simulink model "Working_Shard"  (R2020b)
settings: Solver=VariableStepAuto  StartTime=0.0  StopTime=200  RelTol=1e-3
values from neighbouring files (symbols this model uses):
  A_2 = [0  0  0; 0  0  0; 0  0  0]    [Angular_gust.mat]    (also in Linear_gust.mat; Real_Values.m = zeros(3); Trial_Script.m = zeros(3); TryingNewAeroCoeffs.m = zeros(3))
  A_AD = [0 0 0 0 0 0 0 0 0 0 0 0 ... (36 elements, 6x6)]    [Angular_gust.mat]    (also in Linear_gust.mat; Real_Values.m = horzcat(A_i, A_ii); Trial_Script.m = horzcat(A_i, A_ii); TryingNewAeroCoeffs.m = horzcat(A_i, A_ii))
  A_kal = [0 0 0 0 0 0 0 0 0 0 0 0 ... (36 elements, 6x6)]    [Angular_gust.mat]    (also in Linear_gust.mat; Real_Values.m = [0 0 0 1 0 0; Trial_Script.m = [0 0 0 1 0 0; TryingNewAeroCoeffs.m = [0 0 0 1 0 0)
  B_2 = [0.0024294842205  2.57653534931e-06  6.44659625064e-05; 0  -0.000916808772026  -2.10833406567e-07; 0  0  -0.000799328564006]    [Angular_gust.mat]    (also in Linear_gust.mat; Real_Values.m = I_inv; Trial_Script.m = I_inv; TryingNewAeroCoeffs.m = I_inv)
  B_AD = [0 0 0 0 0 0 0 0 0 0 0 0 ... (36 elements, 6x6)]    [Angular_gust.mat]    (also in Linear_gust.mat; Real_Values.m = horzcat(B_i, B_ii); Trial_Script.m = horzcat(B_i, B_ii); TryingNewAeroCoeffs.m = horzcat(B_i, B_ii))
  B_kal = [0 0 0 0 0 0 0 0 0 0 0 0 ... (36 elements, 6x6)]    [Angular_gust.mat]    (also in Linear_gust.mat; Real_Values.m = [0 0 0 0 0 0; Trial_Script.m = [0 0 0 0 0 0; TryingNewAeroCoeffs.m = [0 0 0 0 0 0)
  C_2 = [1  0  0; 0  1  0; 0  0  1]    [Angular_gust.mat]    (also in Linear_gust.mat; Real_Values.m = eye(3); Trial_Script.m = eye(3); TryingNewAeroCoeffs.m = eye(3))
  C_AD = [1 0 0 0 0 0 0 1 0 0 0 0 ... (36 elements, 6x6)]    [Angular_gust.mat]    (also in Linear_gust.mat; Real_Values.m = eye(6); Trial_Script.m = eye(6); TryingNewAeroCoeffs.m = eye(6))
  C_D = 0.6    [Angular_gust.mat]    (also in Linear_gust.mat; Trial_Script.m; TryingNewAeroCoeffs.m)
  C_kal = [1 0 0 0 0 0 0 1 0 0 0 0 ... (36 elements, 6x6)]    [Angular_gust.mat]    (also in Linear_gust.mat; Real_Values.m = eye(6); Trial_Script.m = eye(6); TryingNewAeroCoeffs.m = eye(6))
  D_2 = [0  0  0; 0  0  0; 0  0  0]    [Angular_gust.mat]    (also in Linear_gust.mat; Real_Values.m = zeros(3); Trial_Script.m = zeros(3); TryingNewAeroCoeffs.m = zeros(3))
  D_AD = [0 0 0 0 0 0 0 0 0 0 0 0 ... (36 elements, 6x6)]    [Angular_gust.mat]    (also in Linear_gust.mat; Real_Values.m = zeros(6); Trial_Script.m = zeros(6); TryingNewAeroCoeffs.m = zeros(6))
  D_kal = [0 0 0 0 0 0 0 0 0 0 0 0 ... (36 elements, 6x6)]    [Angular_gust.mat]    (also in Linear_gust.mat; Real_Values.m = zeros(6); Trial_Script.m = zeros(6); TryingNewAeroCoeffs.m = zeros(6))
  delta_time = 0.0178961433409    [Angular_gust.mat]    (also in Linear_gust.mat; Real_Values.m = time/length(xdata); Trial_Script.m = time/length(xdata); TryingNewAeroCoeffs.m = time/length(xdata))
  Fb1_l = -2600    [Angular_gust.mat]    (also in Linear_gust.mat; Real_Values.m; Trial_Script.m; TryingNewAeroCoeffs.m)
  Fb1_u = 2600    [Angular_gust.mat]    (also in Linear_gust.mat; Real_Values.m; Trial_Script.m; TryingNewAeroCoeffs.m)
  Fb2_l = -2600    [Angular_gust.mat]    (also in Linear_gust.mat; Real_Values.m; Trial_Script.m; TryingNewAeroCoeffs.m)
  Fb2_u = 2600    [Angular_gust.mat]    (also in Linear_gust.mat; Real_Values.m; Trial_Script.m; TryingNewAeroCoeffs.m)
  Fb3_l = -3200    [Angular_gust.mat]    (also in Linear_gust.mat; Real_Values.m; Trial_Script.m; TryingNewAeroCoeffs.m)
  Fb3_u = 3200    [Angular_gust.mat]    (also in Linear_gust.mat; Real_Values.m; Trial_Script.m; TryingNewAeroCoeffs.m)
  Fb4_l = -3200    [Angular_gust.mat]    (also in Linear_gust.mat; Real_Values.m; Trial_Script.m; TryingNewAeroCoeffs.m)
  Fb4_u = 3200    [Angular_gust.mat]    (also in Linear_gust.mat; Real_Values.m; Trial_Script.m; TryingNewAeroCoeffs.m)
  Fc1_l = -300    [Angular_gust.mat]    (also in Linear_gust.mat; Real_Values.m = -30000; Trial_Script.m = -3000; TryingNewAeroCoeffs.m)
  Fc1_u = 300    [Angular_gust.mat]    (also in Linear_gust.mat; Real_Values.m = 30000; Trial_Script.m = 3000; TryingNewAeroCoeffs.m)
  Fc2_l = -300    [Angular_gust.mat]    (also in Linear_gust.mat; Real_Values.m = -30000; Trial_Script.m = -3000; TryingNewAeroCoeffs.m)
  Fc2_u = 300    [Angular_gust.mat]    (also in Linear_gust.mat; Real_Values.m = 30000; Trial_Script.m = 3000; TryingNewAeroCoeffs.m)
  Fc3_l = -300    [Angular_gust.mat]    (also in Linear_gust.mat; Real_Values.m = -30000; Trial_Script.m = -3000; TryingNewAeroCoeffs.m)
  Fc3_u = 300    [Angular_gust.mat]    (also in Linear_gust.mat; Real_Values.m = 30000; Trial_Script.m = 3000; TryingNewAeroCoeffs.m)
  Ft1_l = -5600    [Angular_gust.mat]    (also in Linear_gust.mat; Real_Values.m; Trial_Script.m; TryingNewAeroCoeffs.m)
  Ft1_u = 5600    [Angular_gust.mat]    (also in Linear_gust.mat; Real_Values.m; Trial_Script.m; TryingNewAeroCoeffs.m)
  Ft2_l = -5600    [Angular_gust.mat]    (also in Linear_gust.mat; Real_Values.m; Trial_Script.m; TryingNewAeroCoeffs.m)
  Ft2_u = 5600    [Angular_gust.mat]    (also in Linear_gust.mat; Real_Values.m; Trial_Script.m; TryingNewAeroCoeffs.m)
  Ft3_l = -3200    [Angular_gust.mat]    (also in Linear_gust.mat; Real_Values.m; Trial_Script.m; TryingNewAeroCoeffs.m)
  Ft3_u = 3200    [Angular_gust.mat]    (also in Linear_gust.mat; Real_Values.m; Trial_Script.m; TryingNewAeroCoeffs.m)
  Ft4_l = -3200    [Angular_gust.mat]    (also in Linear_gust.mat; Real_Values.m; Trial_Script.m; TryingNewAeroCoeffs.m)
  Ft4_u = 3200    [Angular_gust.mat]    (also in Linear_gust.mat; Real_Values.m; Trial_Script.m; TryingNewAeroCoeffs.m)
  g = 9.81    [Angular_gust.mat]    (also in Linear_gust.mat; Real_Values.m; Trial_Script.m; TryingNewAeroCoeffs.m)
  m = 941.102    [Angular_gust.mat]    (also in Linear_gust.mat; Real_Values.m; Trial_Script.m = 645; TryingNewAeroCoeffs.m)
  r_0 = [0 0 0]    [Angular_gust.mat]    (also in Linear_gust.mat; Real_Values.m = [0;0;0]; Trial_Script.m = [0;0;0]; TryingNewAeroCoeffs.m = [0;0;0])
  r_cgCatia = [0.0401998 0.00180957 -0.293434]    [Angular_gust.mat]    (also in Linear_gust.mat; Real_Values.m = TcgCatia*r_cgCatia; Trial_Script.m = [2; 0; 0]; TryingNewAeroCoeffs.m = TcgCatia*r_cgCatia)
  rho = 1.225    [Angular_gust.mat]    (also in Linear_gust.mat; Real_Values.m; Trial_Script.m; TryingNewAeroCoeffs.m)
  S = 1.8    [Angular_gust.mat]    (also in Linear_gust.mat; Trial_Script.m; TryingNewAeroCoeffs.m)
  t_finalgust = 17.9140394843    [Angular_gust.mat]    (also in Linear_gust.mat; Real_Values.m = time; TryingNewAeroCoeffs.m = time)
  TcgCatia = [1  0  0; 0  -1  0; 0  0  -1]    [Angular_gust.mat]    (also in Linear_gust.mat; Real_Values.m = [1 0 0; Trial_Script.m = [1 0 0; TryingNewAeroCoeffs.m = [1 0 0)
  theta_0 = [0 0 0]    [Angular_gust.mat]    (also in Linear_gust.mat; Real_Values.m = [0;0;0]; Trial_Script.m = [0;0;0]; TryingNewAeroCoeffs.m = [0;0;0])
  time_delay = 0.01    [Angular_gust.mat]    (also in Linear_gust.mat; Real_Values.m = 0.1; Trial_Script.m = 0.1; TryingNewAeroCoeffs.m)
  Tzy_Shard = [6.12323399574e-17  1  1.22464679915e-16; 1  -6.12323399574e-17  -7.49879891331e-33; 0  1.22464679915e-16  -1]    [Angular_gust.mat]    (also in Linear_gust.mat; Real_Values.m = [cos(pi/2) -sin(pi/2) 0; sin(pi/2) cos(pi/2) 0; 0 0 1]*[1 0 ; Trial_Script.m = [cos(pi/2) -sin(pi/2) 0; sin(pi/2) cos(pi/2) 0; 0 0 1]*[1 0 ; TryingNewAeroCoeffs.m = [cos(pi/2) -sin(pi/2) 0; sin(pi/2) cos(pi/2) 0; 0 0 1]*[1 0 )
  u0_final = 23.9559    [Angular_gust.mat]    (also in Linear_gust.mat; Real_Values.m = u_0(length(u_0)); TryingNewAeroCoeffs.m = u_0(length(u_0)))
  u1_final = -0.480858    [Angular_gust.mat]    (also in Linear_gust.mat; Real_Values.m = u_1(length(u_1)); TryingNewAeroCoeffs.m = u_1(length(u_1)))
  u2_final = -0.725589    [Angular_gust.mat]    (also in Linear_gust.mat; Real_Values.m = u_2(length(u_2)); TryingNewAeroCoeffs.m = u_2(length(u_2)))
  u_0 = [24.7775 24.7775 24.7775 24.7775 24.7775 24.7775 24.7775 24.7775 24.7775 24.7775 24.7775 24.7775 ... (1001 elements, 1001x1)]    [Angular_gust.mat]    (also in Linear_gust.mat; Real_Values.m = a(1:d_shard,1); Trial_Script.m = a(1:d_shard,1); TryingNewAeroCoeffs.m = a(1:d_shard,1))
  u_1 = [0.712897 0.712897 0.712897 0.712897 0.712897 0.712897 0.712897 0.712897 0.712897 0.712897 0.712897 0.712897 ... (1001 elements, 1001x1)]    [Angular_gust.mat]    (also in Linear_gust.mat; Real_Values.m = a(1:d_shard,2); Trial_Script.m = a(1:d_shard,2); TryingNewAeroCoeffs.m = a(1:d_shard,2))
  u_2 = [-0.504815 -0.504815 -0.504815 -0.504815 -0.504815 -0.504815 -0.504815 -0.504815 -0.504815 -0.504815 -0.504815 -0.504815 ... (1001 elements, 1001x1)]    [Angular_gust.mat]    (also in Linear_gust.mat; Real_Values.m = a(1:d_shard,3); Trial_Script.m = a(1:d_shard,3); TryingNewAeroCoeffs.m = a(1:d_shard,3))
  v_0 = [0 0 0]    [Angular_gust.mat]    (also in Linear_gust.mat; Real_Values.m = [0;0;0]; Trial_Script.m = [0;0;0]; TryingNewAeroCoeffs.m = [0;0;0])
  ZI_Cx = [4.10002314469 4.10486511138 4.10970707807 4.11454904475 4.11939101144 4.12423297813 4.12907494481 4.1339169115 4.13875887819 4.14360084487 4.14844281156 4.15328477825 ... (65341 elements, 361x181)]    [Angular_gust.mat]    (also in Linear_gust.mat; Real_Values.m = model_Cx(XI_Cx, YI_Cx); Trial_Script.m = model_Cx(XI_Cx, YI_Cx); TryingNewAeroCoeffs.m = model_Cx(XI_Cx, YI_Cx))
  ZI_Cy = [5.10662222372 5.15407485934 5.20152749496 5.24898013059 5.29643276621 5.34388540184 5.39133803746 5.43879067308 5.48624330871 5.53369594433 5.58114857996 5.62860121558 ... (65341 elements, 361x181)]    [Angular_gust.mat]    (also in Linear_gust.mat; Real_Values.m = model_Cy(XI_Cy, YI_Cy); Trial_Script.m = model_Cy(XI_Cy, YI_Cy); TryingNewAeroCoeffs.m = model_Cy(XI_Cy, YI_Cy))
  ZI_Cz = [-10.5947720774 -10.6317912004 -10.6688103235 -10.7058294465 -10.7428485695 -10.7798676926 -10.8168868156 -10.8539059387 -10.8909250617 -10.9279441847 -10.9649633078 -11.0019824308 ... (65341 elements, 361x181)]    [Angular_gust.mat]    (also in Linear_gust.mat; Real_Values.m = model_Cz(XI_Cz, YI_Cz); Trial_Script.m = model_Cz(XI_Cz, YI_Cz); TryingNewAeroCoeffs.m = model_Cz(XI_Cz, YI_Cz))
  ZI_p = [6.05111971338 6.06712776392 6.08313581446 6.099143865 6.11515191553 6.13115996607 6.14716801661 6.16317606715 6.17918411769 6.19519216823 6.21120021877 6.22720826931 ... (65341 elements, 361x181)]    [Angular_gust.mat]    (also in Linear_gust.mat; Real_Values.m = model_p(XI_p, YI_p); Trial_Script.m = model_p(XI_p, YI_p); TryingNewAeroCoeffs.m = model_p(XI_p, YI_p))
  ZI_q = [0.071083987219 0.054175962948 0.0372679386771 0.0203599144061 0.00345189013513 -0.0134561341358 -0.0303641584068 -0.0472721826778 -0.0641802069487 -0.0810882312197 -0.0979962554907 -0.114904279762 ... (65341 elements, 361x181)]    [Angular_gust.mat]    (also in Linear_gust.mat; Real_Values.m = model_q(XI_q, YI_q); Trial_Script.m = model_q(XI_q, YI_q); TryingNewAeroCoeffs.m = model_q(XI_q, YI_q))
  ZI_r = [-1.8762921931 -1.88364224017 -1.89099228723 -1.8983423343 -1.90569238136 -1.91304242842 -1.92039247549 -1.92774252255 -1.93509256961 -1.94244261668 -1.94979266374 -1.95714271081 ... (65341 elements, 361x181)]    [Angular_gust.mat]    (also in Linear_gust.mat; Real_Values.m = model_r(XI_r, YI_r); Trial_Script.m = model_r(XI_r, YI_r); TryingNewAeroCoeffs.m = model_r(XI_r, YI_r))
undefined symbols (not defined in the file or in its folder): Continuous, Time
libraries: dspsigops x11, simulink x7, pid_lib x3, fuzblock x3, dspindex x3, ctrlSharedLib x2, sharedutil x1, mpclib x1, dspmathops x1, cstblocks x1
(part 1 of 2)
settings Model: Creator=Jonathan van Zyl  LastModifiedBy=Jonathan van Zyl

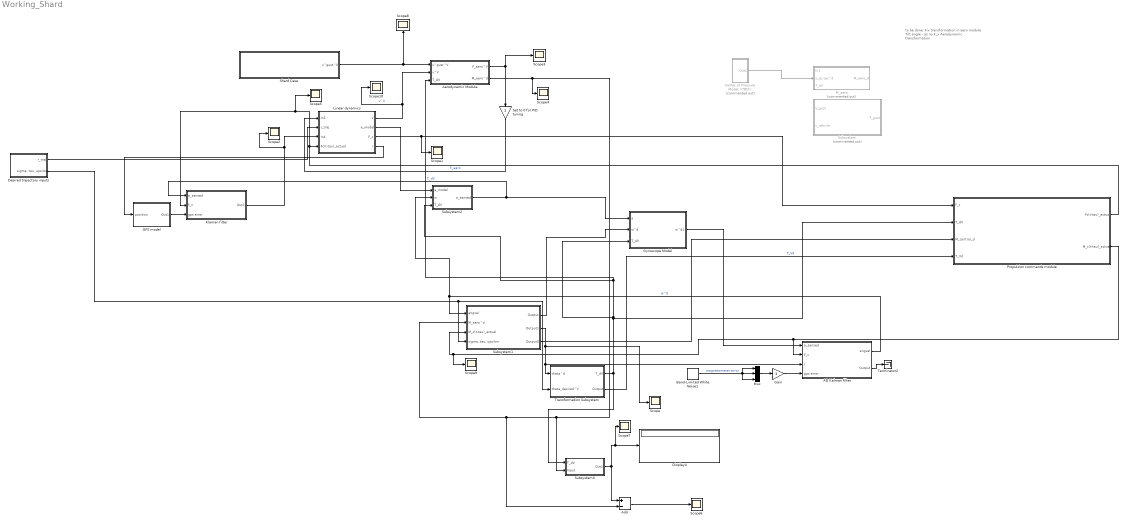
== system Working_Shard ==
  note: to be done:
      | Fix transformation in aero module
      | Tilt angle - as no F_x
      | Aerodynamic transformation
  AD Kalman filter : Subsystem
  Add : Sum  Inputs=+-
  Aerodynamic Module : Subsystem
  Band-Limited White Noise1 : simulink/Sources/Band-Limited White Noise  Cov=[0.000000001]  Ts=0.1  seed=[23341]
  Center of Pressure Model <TBD> : Subsystem  Commented=on
  Desired trajectory inputs : Subsystem
  Display4 : Display
  GPS model : Subsystem
  Gain : Gain
  Gyroscope Model : Subsystem
  Klaman filter : Subsystem
  Linear dynamics : Subsystem
  M_aero : Subsystem  Commented=on
  Mux : Mux  Inputs=3
  Propulsion commands module : Subsystem
  Scope{,1..10} (11 alike) : Scope
  Set to 0 for PID tuning : Gain
  Shard Case : Subsystem
  Subsystem : Subsystem  Commented=on
  Subsystem1 : Subsystem
  Subsystem2 : Subsystem
  Subsystem3 : Subsystem
  Terminator2 : Terminator
  Transformation Subsystem : Subsystem
  wires:
  Propulsion commands module/2(M_c(t-tau)_actual) -> AD Kalman filter/2(F_c), Scope9/1, Subsystem1/3(M_c(t-tau)_actual)
  Linear dynamics/3(F_c) -> Propulsion commands module/1(F_c), Scope1/1
  Gyroscope Model/1(w^d1) -> AD Kalman filter/1(a_sensed)
  GPS model/1(Out1) -> Klaman filter/3(gps error)
  Aerodynamic Module/2(M_aero^d) -> Scope4/1, Add/2, Subsystem1/2(M_aero^d), Subsystem3/2(Input)
  Subsystem3/1(Out1) -> Add/1, Scope7/1, Display4/1
  Shard Case/1(v^gust^V) -> Scope8/1, Aerodynamic Module/1(v^gust^V)
  Add/1 -> Scope6/1
  AD Kalman filter/1(angvel) -> Subsystem2/2(w), Subsystem1/1(angvel)  "w^d"
  Aerodynamic Module/1(F_aero^V) -> Set to 0 for PID tuning/1, Scope3/1
  Subsystem2/1(a_sensed) -> Gyroscope Model/1(a), Klaman filter/1(a_sensed)
  Linear dynamics/2(a_model) -> Subsystem2/1(a_model)
  Center of Pressure Model <TBD>/1(Out1) -> M_aero/2(x_cp vec^d)
  Subsystem1/2(Output1) -> Transformation Subsystem/1(theta^d), AD Kalman filter/3(r), Scope/1
  Transformation Subsystem/1(T_dV) -> Subsystem3/1(T_dV), Aerodynamic Module/3(T_dV), Subsystem2/3(T_dV), Gyroscope Model/3(T_dV), Propulsion commands module/2(T_dV)  "T_dV"
  Subsystem1/1(Output) -> Gyroscope Model/2(w^d)
  AD Kalman filter/2(Output) -> Terminator2/1
  Mux/1 -> Gain/1
  Gain/1 -> AD Kalman filter/4(gps error)
  Desired trajectory inputs/2("sigma, tau, upsilon") -> Transformation Subsystem/2(theta_desired^V), Subsystem1/4("sigma, tau, upsilon")
  Klaman filter/1(Out1) -> Scope2/1, Linear dynamics/3(In4)
  Desired trajectory inputs/1(r_traj) -> Linear dynamics/2(r_traj)
  Band-Limited White Noise1/1 -> Mux/1, Mux/2, Mux/3  "magnetometer error"
  Linear dynamics/1(v) -> Scope10/1, Aerodynamic Module/2(v^V)  "v^V"
  Subsystem1/3(Output3) -> Propulsion commands module/3(M_control_d)
  Linear dynamics/4(r) -> GPS model/1(position)
  Set to 0 for PID tuning/1 -> Linear dynamics/1(In1)  "F_aero"
  Propulsion commands module/1(Fc(t-tau)_actual) -> Scope5/1, Klaman filter/2(F_c), Linear dynamics/4(Fc(t-tau)_actual)
  Transformation Subsystem/2(Output) -> Propulsion commands module/4(T_Vd)  "T_Vd"

== system Working_Shard/AD Kalman filter ==
  a_sensed : Inport
  F_c : Inport  Port=2
  r : Inport  Port=3
  gps error : Inport  Port=4
  Add : Sum
  Constant4 : Constant  Value=0
  Demux1 : Demux  Outputs=6
  Gain4 : Gain
  Kalman Filter : ctrlSharedLib/Kalman Filter  TimeDomain=Continuous-Time  UseCurrentEstimator=on  ModelSource=Individual A, B, C, D matrices  ModelSourceVariable=ss(0.95,1,1,0,1)  A=A_AD  B=B_AD  C=C_AD  D=D_AD  NumberOfStates=1  NumberOfInputs=1  NumberOfOutputs=1  InitialEstimateSource=Dialog  X0=[0;0;0;0;0;0]  P0=10  UseK=off  UseGH=off  NumberOfProcessNoiseInputs=1  G=1  TimeInvariantG=on  H=0  TimeInvariantH=on  Q=0.05  TimeInvariantQ=on  R=1  TimeInvariantR=on  N=0  TimeInvariantN=on  AddInputPort=on  AddEnablePort=off  OutputEstimatedY=off  OutputP=off  Ts=-1
  Mux : Mux  Inputs=3
  Mux1 : Mux
  Mux2 : Mux  Inputs=2
  Mux3 : Mux  Inputs=3
  Scope1 : Scope
  angvel : Outport
  Output : Outport  Port=2
  wires:
  Demux1/5 -> Mux/2
  Mux2/1 -> Kalman Filter/2
  Constant4/1 -> Mux1/3, Mux1/1, Mux1/2
  gps error/1 -> Gain4/1  "theta_error"
  r/1 -> Scope1/1, Add/1  "theta_model"
  Demux1/4 -> Mux/1
  Demux1/2 -> Mux3/2
  Mux1/1 -> Kalman Filter/1
  F_c/1 -> Mux1/4  "Control Torques"
  Demux1/1 -> Mux3/1
  Kalman Filter/1 -> Demux1/1
  Demux1/6 -> Mux/3
  Gain4/1 -> Add/2
  Demux1/3 -> Mux3/3
  Add/1 -> Mux2/1  "theta_sensed"
  Mux3/1 -> angvel/1  "w_kalman"
  a_sensed/1 -> Mux2/2  "sensed angular velocity"
  Mux/1 -> Output/1  "wdot_kalman"

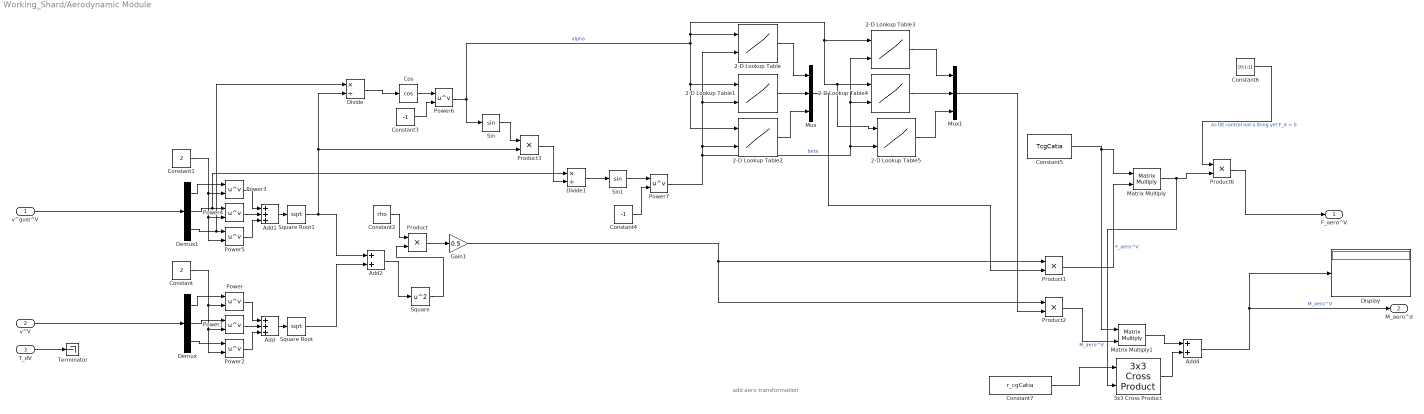
== system Working_Shard/Aerodynamic Module ==
  note: add aero transformation
  v^gust^V : Inport
  v^V : Inport  Port=2
  T_dV : Inport  Port=3
  2-D Lookup Table : Lookup_n-D  BreakpointsForDimension1=[-180:1:180]  BreakpointsForDimension2=[-180:1:180]  Table=ZI_Cx  InternalRulePriority=Speed  RndMeth=Simplest  InputSameDT=on
      settings: InputPortMap=u0,u1
  2-D Lookup Table1 : Lookup_n-D  BreakpointsForDimension1=[-180:1:180]  BreakpointsForDimension2=[-180:1:180]  Table=ZI_Cy  InternalRulePriority=Speed  RndMeth=Simplest  InputSameDT=on
      settings: InputPortMap=u0,u1
  2-D Lookup Table2 : Lookup_n-D  BreakpointsForDimension1=[-180:1:180]  BreakpointsForDimension2=[-180:1:180]  Table=ZI_Cz  InternalRulePriority=Speed  RndMeth=Simplest  InputSameDT=on
      settings: InputPortMap=u0,u1
  2-D Lookup Table3 : Lookup_n-D  BreakpointsForDimension1=[-180:1:180]  BreakpointsForDimension2=[-180:1:180]  Table=ZI_p  InternalRulePriority=Speed  RndMeth=Simplest  InputSameDT=on
      settings: InputPortMap=u0,u1
  2-D Lookup Table4 : Lookup_n-D  BreakpointsForDimension1=[-180:1:180]  BreakpointsForDimension2=[-180:1:180]  Table=ZI_q  InternalRulePriority=Speed  RndMeth=Simplest  InputSameDT=on
      settings: InputPortMap=u0,u1
  2-D Lookup Table5 : Lookup_n-D  BreakpointsForDimension1=[-180:1:180]  BreakpointsForDimension2=[-180:1:180]  Table=ZI_r  InternalRulePriority=Speed  RndMeth=Simplest  InputSameDT=on
      settings: InputPortMap=u0,u1
  3x3 Cross Product : sharedutil/3x3 Cross Product  aMode=aMode
      settings: SourceProductBaseCode=AE,PW,MT,UV,VE,VP
  Add : Sum  Inputs=+++
  Add1 : Sum  Inputs=+++
  Add2 : Sum
  Add4 : Sum
  Constant : Constant  Value=2
  Constant1 : Constant  Value=2
  Constant2 : Constant  Value=rho
  Constant3 : Constant  Value=-1
  Constant4 : Constant  Value=-1
  Constant5 : Constant  Value=TcgCatia
  Constant6 : Constant  Value=[0;1;1]
  Constant7 : Constant  Value=r_cgCatia
  Cos : Trigonometry  Operator=cos
  Demux : Demux  Outputs=3
  Demux1 : Demux  Outputs=3
  Display : Display
  Divide : Product  Inputs=*/
  Divide1 : Product  Inputs=*/
  Gain1 : Gain  Gain=0.5
  Matrix Multiply : Product  Multiplication=Matrix(*)
  Matrix Multiply1 : Product  Multiplication=Matrix(*)
  Mux : Mux  Inputs=3
  Mux1 : Mux  Inputs=3
  Power{,1..7} (8 alike) : Math  Operator=pow  SaturateOnIntegerOverflow=on
  Product{,1..3,6} (5 alike) : Product
  Sin : Trigonometry
  Sin1 : Trigonometry
  Square : Math  Operator=square  SaturateOnIntegerOverflow=on
  Square Root : Sqrt  SaturateOnIntegerOverflow=on
  Square Root1 : Sqrt  SaturateOnIntegerOverflow=on
  Terminator : Terminator
  F_aero^V : Outport
  M_aero^d : Outport  Port=2
  wires:
  Constant1/1 -> Power5/2, Power4/2, Power3/2
  Product1/1 -> Matrix Multiply/2  "F_aero^V"
  Square Root/1 -> Add2/2
  Power6/1 -> Sin/1, 2-D Lookup Table/1, 2-D Lookup Table5/1, 2-D Lookup Table4/1, 2-D Lookup Table3/1, 2-D Lookup Table2/1, 2-D Lookup Table1/1  "alpha"
  Power1/1 -> Add/2
  2-D Lookup Table5/1 -> Mux1/3
  Constant/1 -> Power2/2, Power1/2, Power/2
  Divide/1 -> Cos/1
  Demux/1 -> Power/1
  Power5/1 -> Add1/3
  2-D Lookup Table/1 -> Mux/1
  Divide1/1 -> Sin1/1
  Demux1/1 -> Power3/1
  Add2/1 -> Square/1
  Add4/1 -> Display/1, M_aero^d/1  "M_aero^V"
  Demux/3 -> Power2/1
  Constant4/1 -> Power7/2
  2-D Lookup Table4/1 -> Mux1/2
  Gain1/1 -> Product2/1, Product1/1
  Constant3/1 -> Power6/2
  Power7/1 -> 2-D Lookup Table/2, 2-D Lookup Table1/2, 2-D Lookup Table2/2, 2-D Lookup Table3/2, 2-D Lookup Table4/2, 2-D Lookup Table5/2  "beta"
  Cos/1 -> Power6/1
  Demux1/3 -> Divide/1, Power5/1
  Product/1 -> Gain1/1
  Sin1/1 -> Power7/1
  Power2/1 -> Add/3
  Sin/1 -> Product3/1
  Mux1/1 -> Product2/2
  Demux1/2 -> Divide1/1, Power4/1
  Power4/1 -> Add1/2
  Add/1 -> Square Root/1
  Power/1 -> Add/1
  Square Root1/1 -> Product3/2, Divide/2, Add2/1
  v^gust^V/1 -> Demux1/1
  2-D Lookup Table3/1 -> Mux1/1
  2-D Lookup Table1/1 -> Mux/2
  Power3/1 -> Add1/1
  Mux/1 -> Product1/2
  Product3/1 -> Divide1/2
  2-D Lookup Table2/1 -> Mux/3
  Add1/1 -> Square Root1/1
  Constant2/1 -> Product/1
  Demux/2 -> Power1/1
  v^V/1 -> Demux/1
  Square/1 -> Product/2
  Constant6/1 -> Product6/1  "As tilt control not a thing yet F_X = 0"
  Product6/1 -> F_aero^V/1
  T_dV/1 -> Terminator/1
  Constant5/1 -> Matrix Multiply1/1, Matrix Multiply/1
  Matrix Multiply/1 -> 3x3 Cross Product/2, Product6/2
  Constant7/1 -> 3x3 Cross Product/1
  Matrix Multiply1/1 -> Add4/1
  3x3 Cross Product/1 -> Add4/2
  Product2/1 -> Matrix Multiply1/2  "M_aero^V"

== system Working_Shard/Center of Pressure Model <TBD> ==
  Constant1 : Constant  Value=[0.1;0.2; 0.05]
  Out1 : Outport
  wires:
  Constant1/1 -> Out1/1  "x_cp"

== system Working_Shard/Desired trajectory inputs ==
  Constant2 : Constant  Value=[0;0; 0]
  Constant3 : Constant  Value=[0;0;0]
  r_traj : Outport
  "sigma, tau, upsilon" : Outport  Port=2
  wires:
  Constant2/1 -> r_traj/1  "r_traj"
  Constant3/1 -> "sigma, tau, upsilon"/1  "sigma, tau, upsilon"

== system Working_Shard/GPS model ==
  position : Inport
  GPS Model : MATLAB Function  TreatAsAtomicUnit=on
  Transpose : Math  Operator=transpose  SaturateOnIntegerOverflow=on
  Out1 : Outport
  wires:
  GPS Model/1(newposition) -> Transpose/1  "gps error"
  position/1 -> GPS Model/1(position)
  Transpose/1 -> Out1/1  "r_sensed"

== system Working_Shard/Gyroscope Model ==
  a : Inport
  w^d : Inport  Port=2
  T_dV : Inport  Port=3
  Demux : Demux  Outputs=3
  MATLAB Function : MATLAB Function  TreatAsAtomicUnit=on
  Terminator : Terminator
  Transpose : Math  Operator=transpose  SaturateOnIntegerOverflow=on
  Transpose2 : Math  Operator=transpose  SaturateOnIntegerOverflow=on
  w^d1 : Outport
  wires:
  T_dV/1 -> Terminator/1
  Transpose2/1 -> w^d1/1
  MATLAB Function/1(gyroData) -> Transpose2/1
  a/1 -> Transpose/1
  Transpose/1 -> MATLAB Function/4(acc)
  w^d/1 -> Demux/1
  Demux/1 -> MATLAB Function/1(xvel)
  Demux/2 -> MATLAB Function/2(yvel)
  Demux/3 -> MATLAB Function/3(zvel)

== system Working_Shard/Klaman filter ==
  a_sensed : Inport
  F_c : Inport  Port=2
  gps error : Inport  Port=3
  Constant4 : Constant  Value=0
  Demux1 : Demux  Outputs=6
  Integrator : Integrator  InitialCondition=v_0
  Kalman Filter : ctrlSharedLib/Kalman Filter  TimeDomain=Continuous-Time  UseCurrentEstimator=on  ModelSource=Individual A, B, C, D matrices  ModelSourceVariable=ss(0.95,1,1,0,1)  A=A_kal  B=B_kal  C=C_kal  D=D_kal  NumberOfStates=1  NumberOfInputs=1  NumberOfOutputs=1  InitialEstimateSource=Dialog  X0=[0;0;0;0;0;0]  P0=10  UseK=off  UseGH=off  NumberOfProcessNoiseInputs=1  G=1  TimeInvariantG=on  H=0  TimeInvariantH=on  Q=0.05  TimeInvariantQ=on  R=1  TimeInvariantR=on  N=0  TimeInvariantN=on  AddInputPort=on  AddEnablePort=off  OutputEstimatedY=off  OutputP=off  Ts=-1
  Mux1 : Mux
  Mux2 : Mux  Inputs=2
  Mux3 : Mux  Inputs=3
  Terminator : Terminator
  Terminator1 : Terminator
  Terminator2 : Terminator
  Out1 : Outport
  wires:
  Demux1/5 -> Terminator1/1
  Mux2/1 -> Kalman Filter/2
  Constant4/1 -> Mux1/3, Mux1/1, Mux1/2
  Demux1/4 -> Terminator/1
  Demux1/2 -> Mux3/2
  Mux1/1 -> Kalman Filter/1
  F_c/1 -> Mux1/4  "Control Force"
  Demux1/1 -> Mux3/1
  Kalman Filter/1 -> Demux1/1
  Demux1/6 -> Terminator2/1
  Demux1/3 -> Mux3/3
  Integrator/1 -> Mux2/2  "v_sensed"
  gps error/1 -> Mux2/1  "r_sensed"
  Mux3/1 -> Out1/1  "r_kalman"
  a_sensed/1 -> Integrator/1  "sensed acceleration"

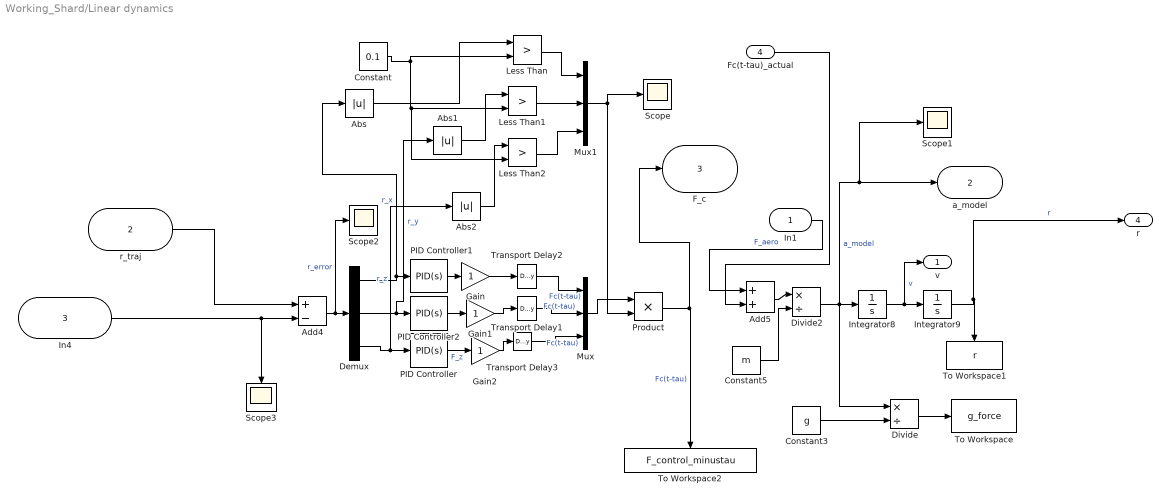
== system Working_Shard/Linear dynamics ==
  In1 : Inport
  r_traj : Inport  Port=2
  In4 : Inport  Port=3
  Fc(t-tau)_actual : Inport  Port=4
  Abs : Abs
  Abs1 : Abs
  Abs2 : Abs
  Add4 : Sum  Inputs=+-
  Add5 : Sum
  Constant : Constant  Value=0.1
  Constant3 : Constant  Value=g
  Constant5 : Constant  Value=m
  Demux : Demux  Outputs=3
  Divide : Product  Inputs=*/
  Divide2 : Product  Inputs=*/
  Gain : Gain
  Gain1 : Gain
  Gain2 : Gain
  Integrator8 : Integrator  InitialCondition=[0;0;0]
  Integrator9 : Integrator  InitialCondition=r_0
  Less Than : RelationalOperator  Operator=>  OutDataTypeStr=boolean  RndMeth=Simplest
  Less Than1 : RelationalOperator  Operator=>  OutDataTypeStr=boolean  RndMeth=Simplest
  Less Than2 : RelationalOperator  Operator=>  OutDataTypeStr=boolean  RndMeth=Simplest
  Mux : Mux  Inputs=3
  Mux1 : Mux  Inputs=3
  PID Controller : pid_lib/PID Controller  Controller=PID  Form=Parallel  TimeDomain=Continuous-time  UseExternalTs=off  SampleTime=-1  IntegratorMethod=Forward Euler  FilterMethod=Forward Euler  ControllerParametersSource=internal  P=9009.63914576468  I=3464.3602040453  D=5659.73322598295  UseFilter=on  N=27.0214258529072  TunerSelectOption=Transfer Function Based (PID Tuner App)  InitialConditionSource=internal  InitialConditionForIntegrator=0  InitialConditionForFilter=0  DifferentiatorICPrevScaledInput=0  ExternalReset=none  TrackingMode=off  Kt=1  LimitOutput=off  SatLimitsSource=internal  UpperSaturationLimit=inf  LowerSaturationLimit=-inf  LinearizeAsGain=on  AntiWindupMode=none  Kb=1  POutMin=[]  POutMax=[]  IOutMin=[]  IOutMax=[]  DOutMin=[]  DOutMax=[]  NOutMin=[]  NOutMax=[]  SumOutMin=[]  SumOutMax=[]  SaturationOutMin=[]  SaturationOutMax=[]  PParamMin=[]  PParamMax=[]  IParamMin=[]  IParamMax=[]  DParamMin=[]  DParamMax=[]  NParamMin=[]  NParamMax=[]  KbParamMin=[]  KbParamMax=[]  KtParamMin=[]  KtParamMax=[]  KbOutMin=[]  KbOutMax=[]  KtOutMin=[]  KtOutMax=[]  IntegratorOutMin=[]  IntegratorOutMax=[]  FilterOutMin=[]  FilterOutMax=[]  SumI1OutMin=[]  SumI1OutMax=[]  SumI2OutMin=[]  SumI2OutMax=[]  SumI3OutMin=[]  SumI3OutMax=[]  SumI4OutMin=[]  SumI4OutMax=[]  SumDOutMin=[]  SumDOutMax=[]  DifferentiatorOutMin=[]  DifferentiatorOutMax=[]  FilterDiffOutCoefMin=[]  FilterDiffOutCoefMax=[]  ReciprocalOutMin=[]  ReciprocalOutMax=[]  SumDenOutMin=[]  SumDenOutMax=[]  SumNumOutMin=[]  SumNumOutMax=[]  DivideOutMin=[]  DivideOutMax=[]  UdiffTsProdOutMin=[]  UdiffTsProdOutMax=[]  NTsProdOutMin=[]  NTsProdOutMax=[]  UintegralTsProdOutMin=[]  UintegralTsProdOutMax=[]  UngainTsProdOutMin=[]  UngainTsProdOutMax=[]  IntegratorContinuousStateAttributes=''  IntegratorStateMustResolveToSignalObject=off  IntegratorRTWStateStorageClass=Auto  FilterContinuousStateAttributes=''  FilterStateMustResolveToSignalObject=off  FilterRTWStateStorageClass=Auto  ParallelPVariant=InternalParameters  IdealPVariant=Disabled  IVariant=InternalParameters  DVariant=InternalParameters  IntegratorVariant=Continuous  SatVariant=Disabled  AWVariant=Passthrough  PCopyVariant=Disabled  TRVariant=Disabled  FdbkBlocksVariant=Forward  IdealPFdbkVariant=Disabled  SatFdbkVariant=Disabled  DerivativeFilterVariant=ContFilter  NVariant=InternalParameters  NCopyVariant=Disabled  FilterICVariant=InternalICsFilter  IntegratorICVariant=InternalICs  ExternalResetVariant=Disabled  TRSumVariant=Passthrough  SumFdbkVariant=Disabled  SumVariant=Sum_PID  TsampFilterVariant=InternalTs  TsampNgainVariant=Passthrough  TsampIntegralVariant=Passthrough  ExternalSaturationOutDataTypeStr=Inherit: Same as second input
  PID Controller1 : pid_lib/PID Controller  Controller=PID  Form=Parallel  TimeDomain=Continuous-time  UseExternalTs=off  SampleTime=-1  IntegratorMethod=Forward Euler  FilterMethod=Forward Euler  ControllerParametersSource=internal  P=9009.63914576468  I=3464.36020404063  D=5659.73322596604  UseFilter=on  N=27.0214258528983  TunerSelectOption=Transfer Function Based (PID Tuner App)  InitialConditionSource=internal  InitialConditionForIntegrator=0  InitialConditionForFilter=0  DifferentiatorICPrevScaledInput=0  ExternalReset=none  TrackingMode=off  Kt=1  LimitOutput=off  SatLimitsSource=internal  UpperSaturationLimit=inf  LowerSaturationLimit=-inf  LinearizeAsGain=on  AntiWindupMode=none  Kb=1  POutMin=[]  POutMax=[]  IOutMin=[]  IOutMax=[]  DOutMin=[]  DOutMax=[]  NOutMin=[]  NOutMax=[]  SumOutMin=[]  SumOutMax=[]  SaturationOutMin=[]  SaturationOutMax=[]  PParamMin=[]  PParamMax=[]  IParamMin=[]  IParamMax=[]  DParamMin=[]  DParamMax=[]  NParamMin=[]  NParamMax=[]  KbParamMin=[]  KbParamMax=[]  KtParamMin=[]  KtParamMax=[]  KbOutMin=[]  KbOutMax=[]  KtOutMin=[]  KtOutMax=[]  IntegratorOutMin=[]  IntegratorOutMax=[]  FilterOutMin=[]  FilterOutMax=[]  SumI1OutMin=[]  SumI1OutMax=[]  SumI2OutMin=[]  SumI2OutMax=[]  SumI3OutMin=[]  SumI3OutMax=[]  SumI4OutMin=[]  SumI4OutMax=[]  SumDOutMin=[]  SumDOutMax=[]  DifferentiatorOutMin=[]  DifferentiatorOutMax=[]  FilterDiffOutCoefMin=[]  FilterDiffOutCoefMax=[]  ReciprocalOutMin=[]  ReciprocalOutMax=[]  SumDenOutMin=[]  SumDenOutMax=[]  SumNumOutMin=[]  SumNumOutMax=[]  DivideOutMin=[]  DivideOutMax=[]  UdiffTsProdOutMin=[]  UdiffTsProdOutMax=[]  NTsProdOutMin=[]  NTsProdOutMax=[]  UintegralTsProdOutMin=[]  UintegralTsProdOutMax=[]  UngainTsProdOutMin=[]  UngainTsProdOutMax=[]  IntegratorContinuousStateAttributes=''  IntegratorStateMustResolveToSignalObject=off  IntegratorRTWStateStorageClass=Auto  FilterContinuousStateAttributes=''  FilterStateMustResolveToSignalObject=off  FilterRTWStateStorageClass=Auto  ParallelPVariant=InternalParameters  IdealPVariant=Disabled  IVariant=InternalParameters  DVariant=InternalParameters  IntegratorVariant=Continuous  SatVariant=Disabled  AWVariant=Passthrough  PCopyVariant=Disabled  TRVariant=Disabled  FdbkBlocksVariant=Forward  IdealPFdbkVariant=Disabled  SatFdbkVariant=Disabled  DerivativeFilterVariant=ContFilter  NVariant=InternalParameters  NCopyVariant=Disabled  FilterICVariant=InternalICsFilter  IntegratorICVariant=InternalICs  ExternalResetVariant=Disabled  TRSumVariant=Passthrough  SumFdbkVariant=Disabled  SumVariant=Sum_PID  TsampFilterVariant=InternalTs  TsampNgainVariant=Passthrough  TsampIntegralVariant=Passthrough  ExternalSaturationOutDataTypeStr=Inherit: Same as second input
  PID Controller2 : pid_lib/PID Controller  Controller=PID  Form=Parallel  TimeDomain=Continuous-time  UseExternalTs=off  SampleTime=-1  IntegratorMethod=Forward Euler  FilterMethod=Forward Euler  ControllerParametersSource=internal  P=9009.63914576468  I=3464.36020397681  D=5659.73322587286  UseFilter=on  N=27.0214258527793  TunerSelectOption=Transfer Function Based (PID Tuner App)  InitialConditionSource=internal  InitialConditionForIntegrator=0  InitialConditionForFilter=0  DifferentiatorICPrevScaledInput=0  ExternalReset=none  TrackingMode=off  Kt=1  LimitOutput=off  SatLimitsSource=internal  UpperSaturationLimit=inf  LowerSaturationLimit=-inf  LinearizeAsGain=on  AntiWindupMode=none  Kb=1  POutMin=[]  POutMax=[]  IOutMin=[]  IOutMax=[]  DOutMin=[]  DOutMax=[]  NOutMin=[]  NOutMax=[]  SumOutMin=[]  SumOutMax=[]  SaturationOutMin=[]  SaturationOutMax=[]  PParamMin=[]  PParamMax=[]  IParamMin=[]  IParamMax=[]  DParamMin=[]  DParamMax=[]  NParamMin=[]  NParamMax=[]  KbParamMin=[]  KbParamMax=[]  KtParamMin=[]  KtParamMax=[]  KbOutMin=[]  KbOutMax=[]  KtOutMin=[]  KtOutMax=[]  IntegratorOutMin=[]  IntegratorOutMax=[]  FilterOutMin=[]  FilterOutMax=[]  SumI1OutMin=[]  SumI1OutMax=[]  SumI2OutMin=[]  SumI2OutMax=[]  SumI3OutMin=[]  SumI3OutMax=[]  SumI4OutMin=[]  SumI4OutMax=[]  SumDOutMin=[]  SumDOutMax=[]  DifferentiatorOutMin=[]  DifferentiatorOutMax=[]  FilterDiffOutCoefMin=[]  FilterDiffOutCoefMax=[]  ReciprocalOutMin=[]  ReciprocalOutMax=[]  SumDenOutMin=[]  SumDenOutMax=[]  SumNumOutMin=[]  SumNumOutMax=[]  DivideOutMin=[]  DivideOutMax=[]  UdiffTsProdOutMin=[]  UdiffTsProdOutMax=[]  NTsProdOutMin=[]  NTsProdOutMax=[]  UintegralTsProdOutMin=[]  UintegralTsProdOutMax=[]  UngainTsProdOutMin=[]  UngainTsProdOutMax=[]  IntegratorContinuousStateAttributes=''  IntegratorStateMustResolveToSignalObject=off  IntegratorRTWStateStorageClass=Auto  FilterContinuousStateAttributes=''  FilterStateMustResolveToSignalObject=off  FilterRTWStateStorageClass=Auto  ParallelPVariant=InternalParameters  IdealPVariant=Disabled  IVariant=InternalParameters  DVariant=InternalParameters  IntegratorVariant=Continuous  SatVariant=Disabled  AWVariant=Passthrough  PCopyVariant=Disabled  TRVariant=Disabled  FdbkBlocksVariant=Forward  IdealPFdbkVariant=Disabled  SatFdbkVariant=Disabled  DerivativeFilterVariant=ContFilter  NVariant=InternalParameters  NCopyVariant=Disabled  FilterICVariant=InternalICsFilter  IntegratorICVariant=InternalICs  ExternalResetVariant=Disabled  TRSumVariant=Passthrough  SumFdbkVariant=Disabled  SumVariant=Sum_PID  TsampFilterVariant=InternalTs  TsampNgainVariant=Passthrough  TsampIntegralVariant=Passthrough  ExternalSaturationOutDataTypeStr=Inherit: Same as second input
  Product : Product
  Scope{,1..3} (4 alike) : Scope
  To Workspace : ToWorkspace  VariableName=g_force  SaveFormat=Timeseries  SampleTime=-1
      settings: Save2DSignal=2-D array (concatenate along first dimension)
  To Workspace1 : ToWorkspace  VariableName=r  SaveFormat=Timeseries  SampleTime=-1
  To Workspace2 : ToWorkspace  VariableName=F_control_minustau  SaveFormat=Timeseries  SampleTime=-1
  Transport Delay1 : TransportDelay  DelayTime=time_delay  TransDelayFeedthrough=on
  Transport Delay2 : TransportDelay  DelayTime=time_delay  TransDelayFeedthrough=on
  Transport Delay3 : TransportDelay  DelayTime=time_delay  TransDelayFeedthrough=on
  v : Outport
  a_model : Outport  Port=2
  F_c : Outport  Port=3
  r : Outport  Port=4
  wires:
  Divide2/1 -> Divide/1, Scope1/1, a_model/1, Integrator8/1  "a_model"
  In4/1 -> Add4/2, Scope3/1
  Divide/1 -> To Workspace/1
  r_traj/1 -> Add4/1
  PID Controller2/1 -> Gain1/1
  Add5/1 -> Divide2/1
  Constant5/1 -> Divide2/2
  Demux/1 -> Abs/1, PID Controller1/1  "r_x"
  PID Controller/1 -> Gain2/1  "F_z"
  Gain1/1 -> Transport Delay1/1
  Add4/1 -> Scope2/1, Demux/1  "r_error"
  Integrator9/1 -> r/1, To Workspace1/1  "r"
  Demux/2 -> Abs1/1, PID Controller2/1  "r_y"
  Product/1 -> F_c/1, To Workspace2/1  "Fc(t-tau)"
  PID Controller1/1 -> Gain/1
  Constant3/1 -> Divide/2
  Gain/1 -> Transport Delay2/1
  Demux/3 -> Abs2/1, PID Controller/1  "r_z"
  Gain2/1 -> Transport Delay3/1
  Integrator8/1 -> Integrator9/1, v/1  "v"
  In1/1 -> Add5/1  "F_aero"
  Transport Delay2/1 -> Mux/1  "Fc(t-tau)"
  Transport Delay1/1 -> Mux/2  "Fc(t-tau)"
  Transport Delay3/1 -> Mux/3  "Fc(t-tau)"
  Constant/1 -> Less Than2/2, Less Than1/2, Less Than/2
  Less Than1/1 -> Mux1/2
  Less Than/1 -> Mux1/1
  Less Than2/1 -> Mux1/3
  Mux/1 -> Product/1
  Mux1/1 -> Product/2, Scope/1
  Abs/1 -> Less Than/1
  Abs1/1 -> Less Than1/1
  Abs2/1 -> Less Than2/1
  Fc(t-tau)_actual/1 -> Add5/2

== system Working_Shard/M_aero ==
  In1 : Inport
  x_cp vec^d : Inport  Port=2
  T_dV : Inport  Port=3
  Matrix Multiply : Product  Multiplication=Matrix(*)
  Matrix Multiply1 : Product
  M_aero_d : Outport
  wires:
  Matrix Multiply/1 -> Matrix Multiply1/2  "F_dis^d"
  x_cp vec^d/1 -> Matrix Multiply1/1  "x_cp"
  T_dV/1 -> Matrix Multiply/1
  In1/1 -> Matrix Multiply/2  "F_gust"
  Matrix Multiply1/1 -> M_aero_d/1  "M_aero_d"

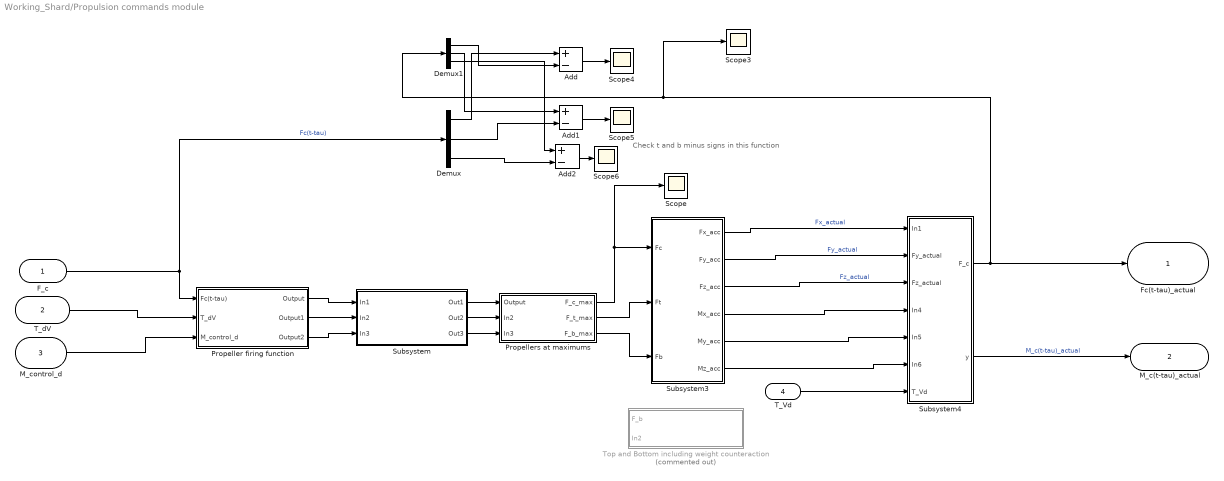
== system Working_Shard/Propulsion commands module ==
  note: Check t and b minus signs in this function
  F_c : Inport
  T_dV : Inport  Port=2
  M_control_d : Inport  Port=3
  T_Vd : Inport  Port=4
  Add : Sum  Inputs=+-
  Add1 : Sum  Inputs=+-
  Add2 : Sum  Inputs=+-
  Demux : Demux  Outputs=3
  Demux1 : Demux  Outputs=3
  Propeller firing function : Subsystem
  Propellers at maximums : Subsystem
  Scope{,3..6} (5 alike) : Scope
  Subsystem : Subsystem
  Subsystem3 : Subsystem
  Subsystem4 : Subsystem
  Top and Bottom including weight counteraction : Subsystem  Commented=on
  Fc(t-tau)_actual : Outport
  M_c(t-tau)_actual : Outport  Port=2
  wires:
  Subsystem3/2(Fy_acc) -> Subsystem4/2(Fy_actual)  "Fy_actual"
  Subsystem4/1(F_c) -> Fc(t-tau)_actual/1, Scope3/1, Demux1/1
  Demux1/3 -> Add2/1
  Subsystem3/3(Fz_acc) -> Subsystem4/3(Fz_actual)  "Fz_actual"
  Demux/2 -> Add1/2
  T_dV/1 -> Propeller firing function/2(T_dV)
  Subsystem3/1(Fx_acc) -> Subsystem4/1(In1)  "Fx_actual"
  Demux1/2 -> Add1/1
  Propellers at maximums/2(F_t_max) -> Subsystem3/2(Ft)
  Demux1/1 -> Add/2
  Subsystem3/5(My_acc) -> Subsystem4/5(In5)
  Subsystem3/6(Mz_acc) -> Subsystem4/6(In6)
  Propellers at maximums/3(F_b_max) -> Subsystem3/3(Fb)
  Demux/3 -> Add2/2
  Subsystem4/2(y) -> M_c(t-tau)_actual/1  "M_c(t-tau)_actual"
  F_c/1 -> Demux/1, Propeller firing function/1(Fc(t-tau))  "Fc(t-tau)"
  T_Vd/1 -> Subsystem4/7(T_Vd)
  Subsystem3/4(Mx_acc) -> Subsystem4/4(In4)
  Add1/1 -> Scope5/1
  Propellers at maximums/1(F_c_max) -> Scope/1, Subsystem3/1(Fc)
  Add2/1 -> Scope6/1
  Demux/1 -> Add/1
  Add/1 -> Scope4/1
  M_control_d/1 -> Propeller firing function/3(M_control_d)
  Propeller firing function/1(Output) -> Subsystem/1(In1)
  Propeller firing function/2(Output1) -> Subsystem/2(In2)
  Propeller firing function/3(Output2) -> Subsystem/3(In3)
  Subsystem/1(Out1) -> Propellers at maximums/1(Output)
  Subsystem/2(Out2) -> Propellers at maximums/2(In2)
  Subsystem/3(Out3) -> Propellers at maximums/3(In3)

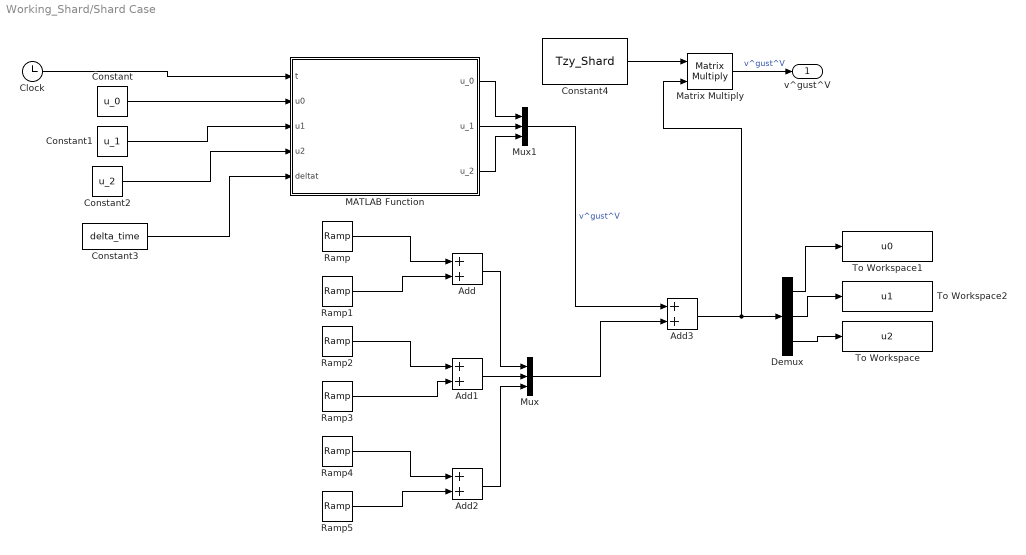
== system Working_Shard/Shard Case ==
  Add{,1..3} (4 alike) : Sum
  Clock : Clock
  Constant : Constant  Value=u_0
  Constant1 : Constant  Value=u_1
  Constant2 : Constant  Value=u_2
  Constant3 : Constant  Value=delta_time
  Constant4 : Constant  Value=Tzy_Shard
  Demux : Demux  Outputs=3
  MATLAB Function : MATLAB Function  TreatAsAtomicUnit=on
  Matrix Multiply : Product  Multiplication=Matrix(*)
  Mux : Mux  Inputs=3
  Mux1 : Mux  Inputs=3
  Ramp : simulink/Sources/Ramp  slope=-1  start=t_finalgust  InitialOutput=0
  Ramp1 : simulink/Sources/Ramp  slope=1  start=t_finalgust + u0_final  InitialOutput=0
  Ramp2 : simulink/Sources/Ramp  slope=-1  start=t_finalgust  InitialOutput=0
  Ramp3 : simulink/Sources/Ramp  slope=1  start=t_finalgust + u1_final  InitialOutput=0
  Ramp4 : simulink/Sources/Ramp  slope=-1  start=t_finalgust  InitialOutput=0
  Ramp5 : simulink/Sources/Ramp  slope=1  start=t_finalgust + u2_final  InitialOutput=0
  To Workspace : ToWorkspace  VariableName=u2  SaveFormat=Timeseries  SampleTime=-1
  To Workspace1 : ToWorkspace  VariableName=u0  SaveFormat=Timeseries  SampleTime=-1
  To Workspace2 : ToWorkspace  VariableName=u1  SaveFormat=Timeseries  SampleTime=-1
  v^gust^V : Outport
  wires:
  Constant2/1 -> MATLAB Function/4(u2)
  Clock/1 -> MATLAB Function/1(t)
  Constant4/1 -> Matrix Multiply/1
  Constant1/1 -> MATLAB Function/3(u1)
  MATLAB Function/2(u_1) -> Mux1/2
  MATLAB Function/3(u_2) -> Mux1/3
  MATLAB Function/1(u_0) -> Mux1/1
  Constant/1 -> MATLAB Function/2(u0)
  Constant3/1 -> MATLAB Function/5(deltat)
  Mux1/1 -> Add3/1  "v^gust^V"
  Matrix Multiply/1 -> v^gust^V/1  "v^gust^V"
  Ramp/1 -> Add/1
  Ramp1/1 -> Add/2
  Ramp3/1 -> Add1/2
  Ramp2/1 -> Add1/1
  Ramp5/1 -> Add2/2
  Ramp4/1 -> Add2/1
  Add/1 -> Mux/1
  Add1/1 -> Mux/2
  Add2/1 -> Mux/3
  Mux/1 -> Add3/2
  Add3/1 -> Demux/1, Matrix Multiply/2
  Demux/2 -> To Workspace2/1
  Demux/3 -> To Workspace/1
  Demux/1 -> To Workspace1/1

== system Working_Shard/Subsystem ==
  V_gust : Inport
  v_vehicle : Inport  Port=2
  Add2 : Sum
  Add3 : Sum
  Drag1 : Subsystem
  Product : Product
  Scope : Scope
  Step2 : Step  Time=0  SampleTime=0
  Step3 : Step  Time=10.5  After=-1  SampleTime=0
  To Workspace : ToWorkspace  VariableName=v_sumsq  SampleTime=-1
  To Workspace1 : ToWorkspace  VariableName=step  SaveFormat=Timeseries  SampleTime=-1
  To Workspace2 : ToWorkspace  VariableName=vtotal  SaveFormat=Timeseries  SampleTime=-1
  To Workspace3 : ToWorkspace  VariableName=F_gust  SaveFormat=Timeseries  SampleTime=-1
  To Workspace4 : ToWorkspace  VariableName=v_gust  SaveFormat=Timeseries  SampleTime=-1
  F_gust : Outport
  wires:
  Product/1 -> F_gust/1, To Workspace3/1, Scope/1  "F_gust"
  Step3/1 -> Add2/1
  V_gust/1 -> To Workspace4/1, Add3/1
  Drag1/1(Out1) -> To Workspace/1
  Add3/1 -> Drag1/1(In1), To Workspace2/1
  Add2/1 -> To Workspace1/1, Product/2
  Step2/1 -> Add2/2
  v_vehicle/1 -> Add3/2
  Drag1/2(drag) -> Product/1

== system Working_Shard/Subsystem1 ==
  angvel : Inport
  M_aero^d : Inport  Port=2
  M_c(t-tau)_actual : Inport  Port=3
  "sigma, tau, upsilon" : Inport  Port=4
  Subsystem : Subsystem
  Output : Outport
  Output1 : Outport  Port=2
  Output3 : Outport  Port=3
  wires:
  M_aero^d/1 -> Subsystem/1(M_aero^d)  "M_aero^d"
  "sigma, tau, upsilon"/1 -> Subsystem/2(Input)  "sigma, tau upsilon"
  Subsystem/1(Output) -> Output1/1  "theta^d"
  Subsystem/2(Output1) -> Output3/1
  Subsystem/3(Out1) -> Output/1
  angvel/1 -> Subsystem/3(angvel)  "angelvel"
  M_c(t-tau)_actual/1 -> Subsystem/4(M_c(t-tau)_actual)

== system Working_Shard/Subsystem2 ==
  a_model : Inport
  w : Inport  Port=2
  T_dV : Inport  Port=3
  Display : Display
  Display1 : Display
  MATLAB Function : MATLAB Function  Commented=on  TreatAsAtomicUnit=on
  Terminator : Terminator
  Terminator3 : Terminator
  Transpose : Math  Operator=transpose  SaturateOnIntegerOverflow=on
  Transpose1 : Math  Operator=transpose  SaturateOnIntegerOverflow=on
  Transpose2 : Math  Operator=transpose  SaturateOnIntegerOverflow=on
  a_sensed : Outport
  wires:
  T_dV/1 -> Terminator3/1
  a_model/1 -> Transpose1/1
  Transpose2/1 -> a_sensed/1  "a_sensed"
  w/1 -> Transpose/1
  Transpose/1 -> Terminator/1
  Transpose1/1 -> Display1/1, Transpose2/1, Display/1  "a_sensed"

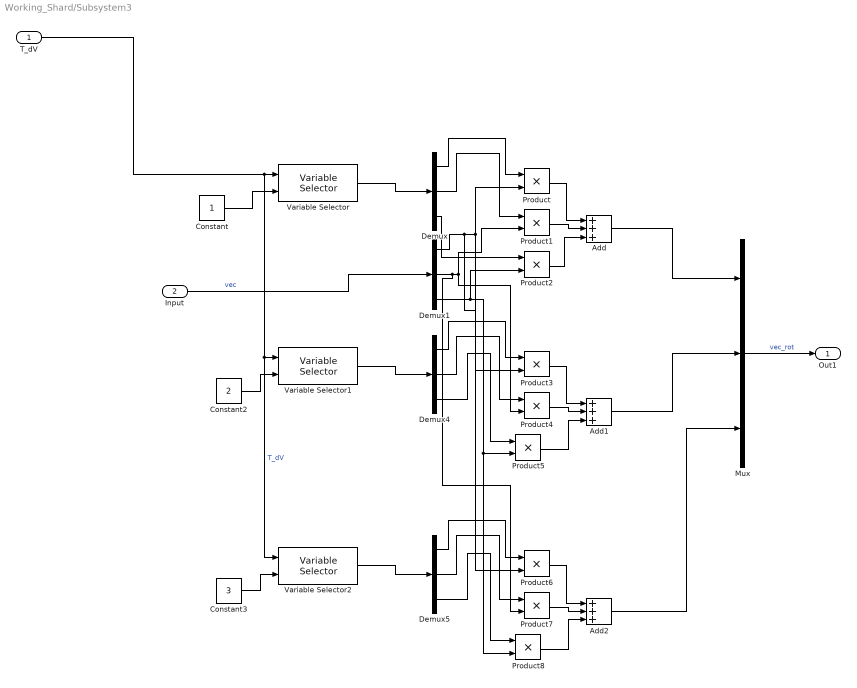
== system Working_Shard/Subsystem3 ==
  T_dV : Inport
  Input : Inport  Port=2
  Add : Sum  Inputs=+++
  Add1 : Sum  Inputs=+++
  Add2 : Sum  Inputs=+++
  Constant : Constant
  Constant2 : Constant  Value=2
  Constant3 : Constant  Value=3
  Demux{,1,4..5} (4 alike) : Demux  Outputs=3
  Mux : Mux  Inputs=3
  Product{,1..8} (9 alike) : Product
  Variable Selector : dspindex/Variable Selector  NumInputs=1  rowsOrCols=Columns  IdxMode=Variable  Elements=[1 3]  ZerOneIdxMode=One-based  errmode=Clip Index  FillMode=on  FillValues=0
  Variable Selector1 : dspindex/Variable Selector  NumInputs=1  rowsOrCols=Columns  IdxMode=Variable  Elements=[1 3]  ZerOneIdxMode=One-based  errmode=Clip Index  FillMode=on  FillValues=0
  Variable Selector2 : dspindex/Variable Selector  NumInputs=1  rowsOrCols=Columns  IdxMode=Variable  Elements=[1 3]  ZerOneIdxMode=One-based  errmode=Clip Index  FillMode=on  FillValues=0
  Out1 : Outport
  wires:
  Variable Selector/1 -> Demux/1
  Add2/1 -> Mux/3
  Demux/1 -> Product/1
  Product3/1 -> Add1/1
  Variable Selector1/1 -> Demux4/1
  Product4/1 -> Add1/2
  Demux4/2 -> Product4/1
  Demux/2 -> Product1/1
  Constant2/1 -> Variable Selector1/2
  Constant/1 -> Variable Selector/2
  Mux/1 -> Out1/1  "vec_rot"
  Add/1 -> Mux/1
  Product5/1 -> Add1/3
  Demux1/2 -> Product7/2, Product1/2, Product4/2
  Product/1 -> Add/1
  Demux5/2 -> Product7/1
  Product8/1 -> Add2/3
  Demux5/3 -> Product8/1
  Product7/1 -> Add2/2
  Demux5/1 -> Product6/1
  Product6/1 -> Add2/1
  Constant3/1 -> Variable Selector2/2
  Demux/3 -> Product2/1
  Variable Selector2/1 -> Demux5/1
  Demux1/3 -> Product8/2, Product5/2, Product2/2
  Product2/1 -> Add/3
  Add1/1 -> Mux/2
  Product1/1 -> Add/2
  Demux4/1 -> Product3/1
  Demux4/3 -> Product5/1
  T_dV/1 -> Variable Selector2/1, Variable Selector1/1, Variable Selector/1  "T_dV"
  Demux1/1 -> Product6/2, Product/2, Product3/2
  Input/1 -> Demux1/1  "vec"

== system Working_Shard/Transformation Subsystem ==
  theta^d : Inport
  theta_desired^V : Inport  Port=2
  Demux2 : Demux  Outputs=3
  Demux3 : Demux  Outputs=3
  Display{,1..3} (4 alike) : Display
  MATLAB Function1 : MATLAB Function  TreatAsAtomicUnit=on
  MATLAB Function2 : MATLAB Function  TreatAsAtomicUnit=on
  Matrix Multiply7 : Product  Multiplication=Matrix(*)
  Terminator{,1..3} (4 alike) : Terminator
  Transpose1 : Math  Operator=transpose  SaturateOnIntegerOverflow=on
  Transpose2 : Math  Operator=transpose  SaturateOnIntegerOverflow=on
  Transpose3 : Math  Operator=transpose  SaturateOnIntegerOverflow=on
  T_dV : Outport
  Output : Outport  Port=2
  wires:
  Demux3/1 -> MATLAB Function1/1(theta_x)
  Demux2/1 -> MATLAB Function2/1(theta_x)
  Transpose2/1 -> Terminator2/1, Matrix Multiply7/2  "T_Vt"
  Demux2/2 -> MATLAB Function2/2(theta_y)
  MATLAB Function2/1(Transformation_Mat) -> Display/1, Terminator/1, Transpose1/1  "T_dt"
  Transpose1/1 -> Terminator1/1, Matrix Multiply7/1  "T_td"
  Demux2/3 -> MATLAB Function2/3(theta_z)
  MATLAB Function1/1(Transformation_Mat) -> Terminator3/1, Transpose2/1  "T_tV"
  Matrix Multiply7/1 -> Display3/1, Output/1, Transpose3/1  "T_Vd"
  theta_desired^V/1 -> Demux3/1
  Demux3/3 -> MATLAB Function1/3(theta_z)
  Demux3/2 -> MATLAB Function1/2(theta_y)
  theta^d/1 -> Display1/1, Demux2/1
  Transpose3/1 -> Display2/1, T_dV/1  "T_dV"

== system Working_Shard/Propulsion commands module/Propeller firing function ==
  Fc(t-tau) : Inport
  T_dV : Inport  Port=2
  M_control_d : Inport  Port=3
  Gain6 : Gain
  MATLAB Function : MATLAB Function  TreatAsAtomicUnit=on
  Matrix Multiply5 : Product  Multiplication=Matrix(*)
  To Workspace : ToWorkspace  VariableName=Fc_wanted  SaveFormat=Timeseries  SampleTime=-1
  To Workspace1 : ToWorkspace  VariableName=Ft_wanted  SaveFormat=Timeseries  SampleTime=-1
  To Workspace2 : ToWorkspace  VariableName=Fb_wanted  SaveFormat=Timeseries  SampleTime=-1
  Turn off for PID tune : Gain
  Output : Outport
  Output1 : Outport  Port=2
  Output2 : Outport  Port=3
  wires:
  Turn off for PID tune/1 -> Matrix Multiply5/2
  Fc(t-tau)/1 -> Turn off for PID tune/1
  Matrix Multiply5/1 -> MATLAB Function/1(F_wanted)  "F_c_d"
  M_control_d/1 -> Gain6/1
  Gain6/1 -> MATLAB Function/2(M_wanted)  "M_c_d"
  MATLAB Function/2(F_t) -> To Workspace1/1, Output1/1  "Ft_wanted"
  MATLAB Function/3(F_b) -> Output2/1, To Workspace2/1  "Fb_wanted"
  MATLAB Function/1(F_c) -> To Workspace/1, Output/1  "Fc_wanted"
  T_dV/1 -> Matrix Multiply5/1

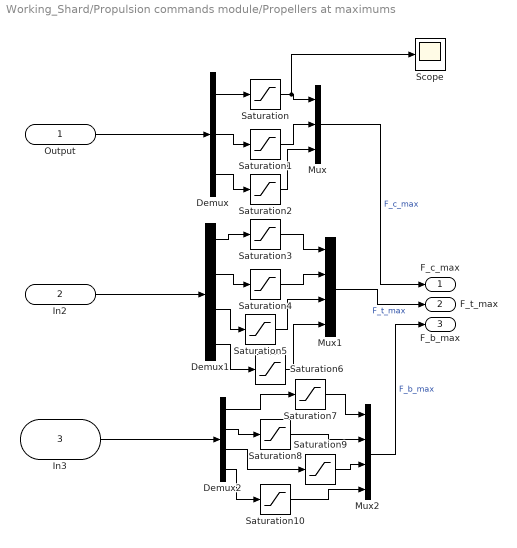
== system Working_Shard/Propulsion commands module/Propellers at maximums ==
  Output : Inport
  In2 : Inport  Port=2
  In3 : Inport  Port=3
  Demux : Demux  Outputs=3
  Demux1 : Demux
  Demux2 : Demux
  Mux : Mux  Inputs=3
  Mux1 : Mux
  Mux2 : Mux
  Saturation : Saturate  UpperLimit=Fc1_u  LowerLimit=Fc1_l
  Saturation1 : Saturate  UpperLimit=Fc2_u  LowerLimit=Fc2_l
  Saturation10 : Saturate  UpperLimit=Fb4_u  LowerLimit=Fb4_l
  Saturation2 : Saturate  UpperLimit=Fc3_u  LowerLimit=Fc3_l
  Saturation3 : Saturate  UpperLimit=Ft1_u  LowerLimit=Ft1_l
  Saturation4 : Saturate  UpperLimit=Ft2_u  LowerLimit=Ft2_l
  Saturation5 : Saturate  UpperLimit=Ft3_u  LowerLimit=Ft3_l
  Saturation6 : Saturate  UpperLimit=Ft4_u  LowerLimit=Ft4_l
  Saturation7 : Saturate  UpperLimit=Fb1_u  LowerLimit=Fb1_l
  Saturation8 : Saturate  UpperLimit=Fb2_u  LowerLimit=Fb2_l
  Saturation9 : Saturate  UpperLimit=Fb3_u  LowerLimit=Fb3_l
  Scope : Scope
  F_c_max : Outport
  F_t_max : Outport  Port=2
  F_b_max : Outport  Port=3
  wires:
  Demux2/1 -> Saturation7/1
  Output/1 -> Demux/1
  Saturation2/1 -> Mux/3
  Mux2/1 -> F_b_max/1  "F_b_max"
  Demux2/2 -> Saturation8/1
  Demux/1 -> Saturation/1
  Demux/2 -> Saturation1/1
  Demux2/3 -> Saturation9/1
  Demux1/1 -> Saturation3/1
  Saturation3/1 -> Mux1/1
  Saturation7/1 -> Mux2/1
  Demux1/4 -> Saturation6/1
  Demux2/4 -> Saturation10/1
  Saturation6/1 -> Mux1/4
  Mux/1 -> F_c_max/1  "F_c_max"
  Saturation/1 -> Scope/1, Mux/1
  Saturation1/1 -> Mux/2
  Mux1/1 -> F_t_max/1  "F_t_max"
  Saturation5/1 -> Mux1/3
  Demux/3 -> Saturation2/1
  Saturation4/1 -> Mux1/2
  Demux1/2 -> Saturation4/1
  Demux1/3 -> Saturation5/1
  Saturation8/1 -> Mux2/2
  Saturation9/1 -> Mux2/3
  Saturation10/1 -> Mux2/4
  In3/1 -> Demux2/1
  In2/1 -> Demux1/1

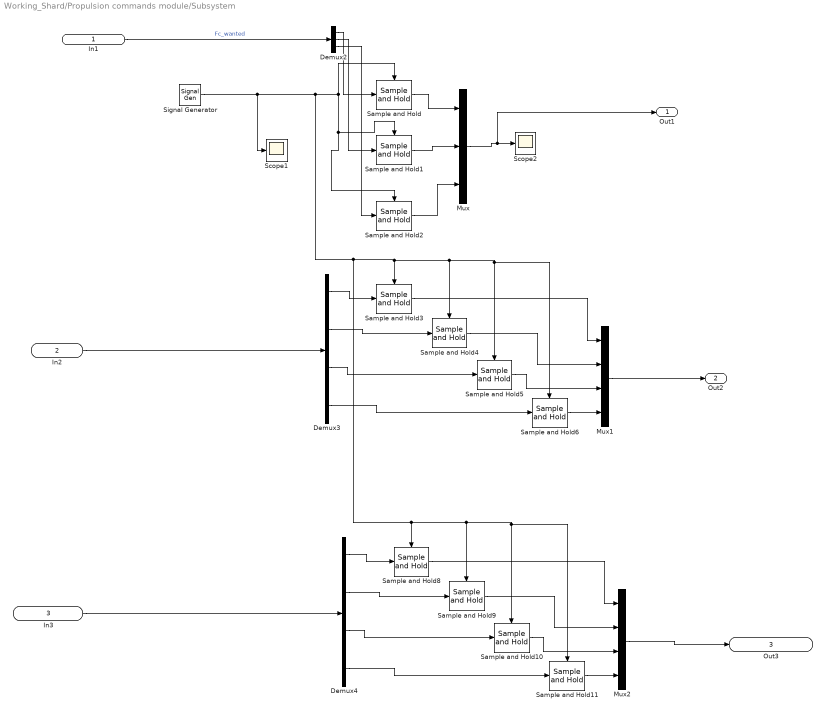
== system Working_Shard/Propulsion commands module/Subsystem ==
  In1 : Inport
  In2 : Inport  Port=2
  In3 : Inport  Port=3
  Demux2 : Demux  Outputs=3
  Demux3 : Demux
  Demux4 : Demux
  Mux : Mux  Inputs=3
  Mux1 : Mux
  Mux2 : Mux
  Sample and Hold{,1..6,8..11} (11 alike) : dspsigops/Sample and Hold  trig=Rising edge  initCond=0  latchinput=off
  Scope1 : Scope
  Scope2 : Scope
  Signal Generator : SignalGenerator  WaveForm=square  Frequency=1000  Units=rad/sec
  Out1 : Outport
  Out2 : Outport  Port=2
  Out3 : Outport  Port=3
  wires:
  Sample and Hold/1 -> Mux/1
  Sample and Hold11/1 -> Mux2/4
  Demux2/2 -> Sample and Hold1/1
  Signal Generator/1 -> Scope1/1, Sample and Hold11/Trigger, Sample and Hold10/Trigger, Sample and Hold9/Trigger, Sample and Hold8/Trigger, Sample and Hold6/Trigger, Sample and Hold5/Trigger, Sample and Hold4/Trigger, Sample and Hold3/Trigger, Sample and Hold/Trigger, Sample and Hold2/Trigger, Sample and Hold1/Trigger
  Demux2/3 -> Sample and Hold2/1
  Sample and Hold8/1 -> Mux2/1
  Sample and Hold1/1 -> Mux/2
  Sample and Hold4/1 -> Mux1/2
  Demux2/1 -> Sample and Hold/1
  In2/1 -> Demux3/1
  Mux/1 -> Out1/1, Scope2/1
  Sample and Hold2/1 -> Mux/3
  Sample and Hold6/1 -> Mux1/4
  Sample and Hold5/1 -> Mux1/3
  Demux3/3 -> Sample and Hold5/1
  Demux3/1 -> Sample and Hold3/1
  Demux3/2 -> Sample and Hold4/1
  Mux2/1 -> Out3/1
  Demux3/4 -> Sample and Hold6/1
  Sample and Hold3/1 -> Mux1/1
  Demux4/2 -> Sample and Hold9/1
  Sample and Hold9/1 -> Mux2/2
  Demux4/1 -> Sample and Hold8/1
  Demux4/4 -> Sample and Hold11/1
  In1/1 -> Demux2/1  "Fc_wanted"
  Demux4/3 -> Sample and Hold10/1
  Sample and Hold10/1 -> Mux2/3
  In3/1 -> Demux4/1
  Mux1/1 -> Out2/1

== system Working_Shard/Propulsion commands module/Subsystem3 ==
  Fc : Inport
  Ft : Inport  Port=2
  Fb : Inport  Port=3
  MATLAB Function : MATLAB Function  TreatAsAtomicUnit=on
  Fx_acc : Outport
  Fy_acc : Outport  Port=2
  Fz_acc : Outport  Port=3
  Mx_acc : Outport  Port=4
  My_acc : Outport  Port=5
  Mz_acc : Outport  Port=6
  wires:
  Fc/1 -> MATLAB Function/1(Fc)
  Ft/1 -> MATLAB Function/2(Ft)
  Fb/1 -> MATLAB Function/3(Fb)
  MATLAB Function/1(Fx_acc) -> Fx_acc/1
  MATLAB Function/2(Fy_acc) -> Fy_acc/1
  MATLAB Function/3(Fz_acc) -> Fz_acc/1
  MATLAB Function/4(Mx_acc) -> Mx_acc/1
  MATLAB Function/5(My_acc) -> My_acc/1
  MATLAB Function/6(Mz_acc) -> Mz_acc/1
